simulink model "invsys"  (Simulink 7.7)
settings: Solver=FixedStepDiscrete  StartTime=0.0  StopTime=200  FixedStep=.001  RelTol=1e-3
values from neighbouring files (symbols this model uses):
  D = [  1 -1  1 -1  1  1 -1 -1 ... (first row only)    [cdma.m]    (also in compressed_sampling.m = idct(eye(5000,5000)))
libraries: simulink x1, dspadpt3 x1, dspsrcs4 x1
settings Model: Creator=Arun  LastModifiedBy=ArunKB

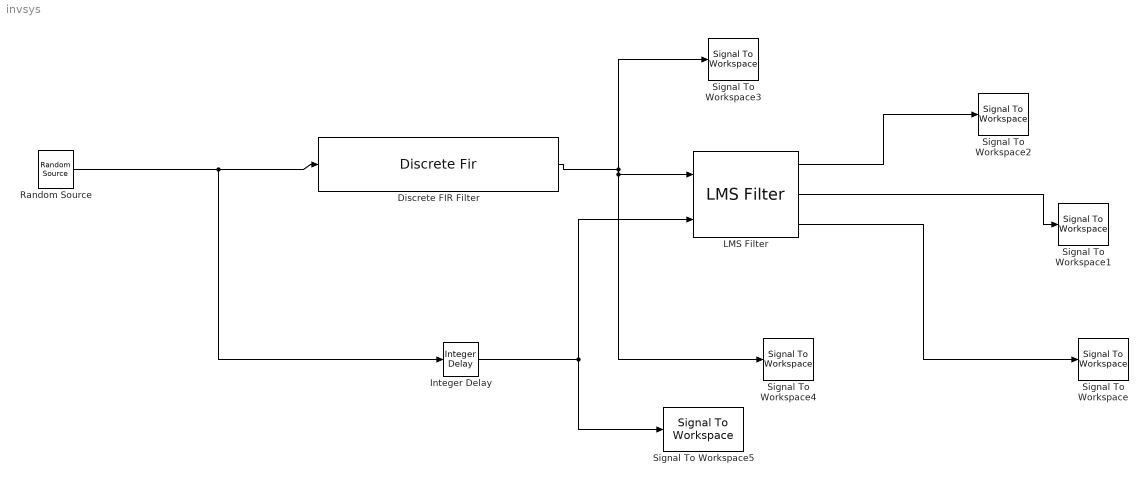
== system invsys ==
  Discrete FIR Filter : DiscreteFir  NumCoeffs=[.1 .4 .5 .2 .9 .7]
  Integer Delay : simulink/Discrete/Integer Delay  NumDelays=16  vinit=0.0  samptime=-1
  LMS Filter : dspadpt3/LMS Filter  Algo=LMS  L=33  stepflag=Dialog  mu=0.01  leakage=1.0  ic=0  Adapt=off  resetflag=None  weights=on  secondCoeffMode=User-defined  secondCoeffWordLength=2  secondCoeffFracLength=15  accum2Mode=User-defined  accum2FracLength=20  prodOutput2Mode=User-defined  prodOutput2FracLength=20  prodOutput3Mode=User-defined  prodOutput3FracLength=20  prodOutput4Mode=User-defined  prodOutput4FracLength=20  quotientMode=User-defined  quotientFracLength=20  roundingMode=Floor  overflowMode=off  addnparflag=off
  Random Source : dspsrcs4/Random Source  SrcType=Gaussian  NormMethod=Ziggurat  CltLength=12  MinVal=0  MaxVal=1  MeanVal=0  VarVal=1  RepMode=Specify seed  rawSeed=88  IsInherit=off  SampMode=Discrete  SampTime=.1  SampFrame=1  DataType=Double  OutComplex=Real
  Signal To Workspace : SignalToWorkspace  VariableName=wts  SaveFormat=Array  Save2DMode=2-D array (concatenate along first dimension)
      settings: CopyFcn=dspblkcopystw(gcbh);  MaxDataPoints=33
  Signal To Workspace1 : SignalToWorkspace  VariableName=error  SaveFormat=Array  Save2DMode=2-D array (concatenate along first dimension)
      settings: CopyFcn=dspblkcopystw(gcbh);
  Signal To Workspace2 : SignalToWorkspace  VariableName=output  SaveFormat=Array  Save2DMode=2-D array (concatenate along first dimension)
      settings: CopyFcn=dspblkcopystw(gcbh);
  Signal To Workspace3 : SignalToWorkspace  VariableName=input  SaveFormat=Array  Save2DMode=2-D array (concatenate along first dimension)
      settings: CopyFcn=dspblkcopystw(gcbh);
  Signal To Workspace4 : SignalToWorkspace  VariableName=filterout  SaveFormat=Array  Save2DMode=2-D array (concatenate along first dimension)
      settings: CopyFcn=dspblkcopystw(gcbh);
  Signal To Workspace5 : SignalToWorkspace  VariableName=delayedout  SaveFormat=Array  Save2DMode=2-D array (concatenate along first dimension)
      settings: CopyFcn=dspblkcopystw(gcbh);
  wires:
  Random Source/1 -> Discrete FIR Filter/1, Integer Delay/1
  LMS Filter/3 -> Signal To Workspace/1
  Discrete FIR Filter/1 -> Signal To Workspace3/1, LMS Filter/1, Signal To Workspace4/1
  Integer Delay/1 -> LMS Filter/2, Signal To Workspace5/1
  LMS Filter/1 -> Signal To Workspace2/1
  LMS Filter/2 -> Signal To Workspace1/1
